simulink model "exercicio2lcsd2"  (R2026a)
settings: Solver=VariableStepAuto

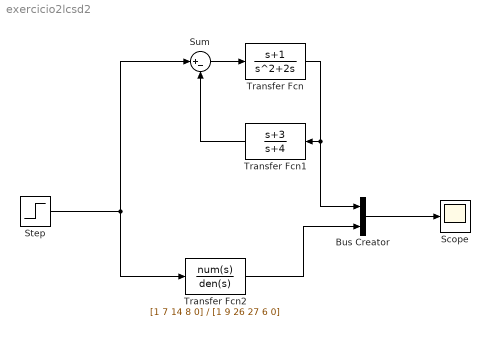
== system exercicio2lcsd2 ==
  Bus Creator : BusCreator  Inputs=2
  Scope : Scope
      settings: ActiveDisplayYMinimum=-0.53241975519524809  ActiveDisplayYMaximum=1.6072735874320596
  Step : Step  SampleTime=0
  Sum : Sum  Inputs=|+-
  Transfer Fcn : TransferFcn  Numerator=[1 1]  Denominator=[1 2 0]
  Transfer Fcn1 : TransferFcn  Numerator=[1 3]  Denominator=[1 4]
  Transfer Fcn2 : TransferFcn  Numerator=[1 7 14 8 0]  Denominator=[1 9 26 27 6 0]
  wires:
  Sum/1 -> Transfer Fcn/1
  Transfer Fcn/1 -> Bus Creator/1, Transfer Fcn1/1
  Transfer Fcn1/1 -> Sum/2
  Step/1 -> Transfer Fcn2/1, Sum/1
  Bus Creator/1 -> Scope/1
  Transfer Fcn2/1 -> Bus Creator/2
